simulink model "ROSCO"  (R2023a)
settings: Solver=ode4  StartTime=0.0  StopTime=TMax  FixedStep=simu.dt  RelTol=1e-3  EnableMultiTasking=on
undefined symbols (not defined in the file): A_total, Azimuth_list, B_total, Bd_total, C_total, D_total, Dd_total, DiscIntNeverNeededParam, F, n_FixFrameInputs, n_FixFrameOutputs, n_FixFrameStates2, n_RotTripletInputs, n_RotTripletOutputs, n_RotTripletStates2, new_seq_inp, new_seq_out, new_seq_states, OutList, Parameter, R, rpm2radps, simu, strmatch, uop_total, windspeed_list, wop_total, xop_total, yop_List_total
libraries: simulink x10
(part 4 of 5)

== matlab function ROSCO/LinearModel_Simulink/Switch op under Azimuth/Switch op under Azimuth ==
  data: Azimuth input; Azimuth_list input; yop_36 input; yop output
function yop  = fcn(Azimuth, Azimuth_list, yop_36)

left = 1;
right = length(Azimuth_list);

while(left<right)
    mid = floor((left + right) / 2);
    if Azimuth_list(mid) == Azimuth
        index = mid;
        break
    elseif Azimuth_list(mid) < Azimuth
        left = mid + 1;
    else
        right = mid - 1;
    end
end
% If target is not found, return the index of the interval in which it falls
if Azimuth < Azimuth_list(1)
    index = 1;
elseif Azimuth > Azimuth_list(end)
    index = length(Azimuth_list);
else
    index = left;
end

yop = yop_36(:, index);
% yop = 1/36 * yop_36(:, 1);
% for i = 2:36
%     yop = yop + 1/36 * yop_36(:, i);
% end

end

== matlab function ROSCO/Monitor2/Cyclic Pitch controller/1P Cyclic Pitch Controller1/Lead Correction ==
  data: bdq input; b_cos output size=1; psi_o input; b_sin output size=1
function [b_cos,b_sin] = fcn(bdq, psi_o)
% This block supports the Embedded MATLAB subset.
% See the help menu for details. 

b_cos=[cosd(psi_o) sind(psi_o)]*bdq;
b_sin=[-sind(psi_o) cosd(psi_o)]*bdq;

== matlab function ROSCO/LinearModel_Simulink/Transverseu/MATLAB Function ==
  data: Azimuth input; n_FixFrameInputs input; n_RotTripletInputs input; delta_u input; new_seq_inp input; delat_u_dq output
function delat_u_dq  = Transverse(Azimuth, n_FixFrameInputs, n_RotTripletInputs, delta_u, new_seq_inp)

% compute azimuth positions of blades:
az = Azimuth*pi/180.0 + 2*pi/3* (0:(3-1)) ; % Eq. 1, azimuth in radians   3个叶片的方位角（弧度），叶片1的方位角为初始方位角

% compute transformation matrices
cos_col = cos(az(:));  % 列向量
sin_col = sin(az(:));

ttv = get_tt_inverse(sin_col, cos_col);     % inverse of tt (computed analytically in function below) 逆矩阵

T1cv = zeros(n_FixFrameInputs+3*n_RotTripletInputs, n_FixFrameInputs+3*n_RotTripletInputs);

T1cv(1:n_FixFrameInputs, 1:n_FixFrameInputs) = eye(n_FixFrameInputs);                % Eq. 21  T1c的逆矩阵

for ii = 1:n_RotTripletInputs
    T1cv(n_FixFrameInputs+1+(ii-1)*3 : n_FixFrameInputs+ii*3, n_FixFrameInputs+1+(ii-1)*3 : n_FixFrameInputs+ii*3) = ttv;
end


% T1o = zeros(n_FixFrameOutputs+3*n_RotTripletOutputs, n_FixFrameOutputs+3*n_RotTripletOutputs);
% 
% T1o(1:n_FixFrameOutputs, 1:n_FixFrameOutputs) = eye(n_FixFrameOutputs);              % Tlo (Eq. 23)  输出相关
% 
% for ii = 1:n_RotTripletOutputs
%     T1o(n_FixFrameOutputs+1+(ii-1)*3 : n_FixFrameOutputs+ii*3, n_FixFrameOutputs+1+(ii-1)*3 : n_FixFrameOutputs+ii*3) = tt;
% end


%% 对u进行转换

delat_u_dq = delta_u .* 0;
delat_u_dq(new_seq_inp, :) = T1cv * delta_u(new_seq_inp);

end



function [ttv] = get_tt_inverse(sin_col, cos_col)

    c1 = cos_col(1);
    c2 = cos_col(2);
    c3 = cos_col(3);
    
    s1 = sin_col(1);
    s2 = sin_col(2);
    s3 = sin_col(3);

    
    ttv = [ c2*s3 - s2*c3,  c3*s1 - s3*c1, c1*s2 - s1*c2
               s2 - s3 ,       s3 - s1,       s1 - s2
               c3 - c2 ,       c1 - c3,       c2 - c1 ] / (1.5*sqrt(3));

    return
end

== matlab function ROSCO/LinearModel_Simulink/Diff of OP ==
  data: Avg_u input; Avg_w input; delta_u output; WindSpeed input; BldPitch input; delta_w output
function [delta_u, delta_w] = fcn(Avg_u, Avg_w, WindSpeed, BldPitch)
    % 相对于工作点的偏差
    delta_u = Avg_u;
    delta_u(1) = BldPitch(1) - Avg_u(1);
    delta_u(2) = BldPitch(2) - Avg_u(2);
    delta_u(3) = BldPitch(3) - Avg_u(3);

    delta_w = Avg_w;
    delta_w(1) = WindSpeed - Avg_w(1);
    % u(9) = BldPitch(1);  
end

== matlab function ROSCO/LinearModel_Simulink/KalmanStateObserver/iMBC ==
  data: Azimuth input; x output; xdq input
function x  = iMBC(Azimuth, xdq)

% compute azimuth positions of blades:
az = Azimuth*pi/180.0 + 2*pi/3* (0:(3-1)) ; % Eq. 1, azimuth in radians   3个叶片的方位角（弧度），叶片1的方位角为初始方位角

% compute transformation matrices
cos_col = cos(az(:));  % 列向量
sin_col = sin(az(:));

tt  = [ones(3,1), cos_col, sin_col];        % Eq. 9, t_tilde

x = xdq .* 0;
x = tt * xdq;

end

== matlab function ROSCO/LinearModel_Simulink/KalmanStateObserver/MBC1 ==
  data: Azimuth input; xdq output; x1 input; x2 input; x3 input
function xdq  = MBC(Azimuth, x1, x2, x3)
x = [x1; x2; x3];
% compute azimuth positions of blades:
az = Azimuth*pi/180.0 + 2*pi/3* (0:(3-1)) ; % Eq. 1, azimuth in radians   3个叶片的方位角（弧度），叶片1的方位角为初始方位角

% compute transformation matrices
cos_col = cos(az(:));  % 列向量
sin_col = sin(az(:));

ttv = get_tt_inverse(sin_col, cos_col);     % inverse of tt (computed analytically in function below) 逆矩阵

xdq = x .* 0;
xdq = ttv * x;

end





function [ttv] = get_tt_inverse(sin_col, cos_col)

    c1 = cos_col(1);
    c2 = cos_col(2);
    c3 = cos_col(3);
    
    s1 = sin_col(1);
    s2 = sin_col(2);
    s3 = sin_col(3);

    
    ttv = [ c2*s3 - s2*c3,  c3*s1 - s3*c1, c1*s2 - s1*c2
               s2 - s3 ,       s3 - s1,       s1 - s2
               c3 - c2 ,       c1 - c3,       c2 - c1 ] / (1.5*sqrt(3));

    return
end

== matlab function ROSCO/LinearModel_Simulink/KalmanStateObserver/MBC2 ==
  data: Azimuth input; xdq output; x1 input; x2 input; x3 input
function xdq  = MBC(Azimuth, x1, x2, x3)
x = [x1; x2; x3];
% compute azimuth positions of blades:
az = Azimuth*pi/180.0 + 2*pi/3* (0:(3-1)) ; % Eq. 1, azimuth in radians   3个叶片的方位角（弧度），叶片1的方位角为初始方位角

% compute transformation matrices
cos_col = cos(az(:));  % 列向量
sin_col = sin(az(:));

ttv = get_tt_inverse(sin_col, cos_col);     % inverse of tt (computed analytically in function below) 逆矩阵

xdq = x .* 0;
xdq = ttv * x;

end





function [ttv] = get_tt_inverse(sin_col, cos_col)

    c1 = cos_col(1);
    c2 = cos_col(2);
    c3 = cos_col(3);
    
    s1 = sin_col(1);
    s2 = sin_col(2);
    s3 = sin_col(3);

    
    ttv = [ c2*s3 - s2*c3,  c3*s1 - s3*c1, c1*s2 - s1*c2
               s2 - s3 ,       s3 - s1,       s1 - s2
               c3 - c2 ,       c1 - c3,       c2 - c1 ] / (1.5*sqrt(3));

    return
end

== matlab function ROSCO/LinearModel_Simulink/KalmanStateObserver/MBC3 ==
  data: Azimuth input; xdq output; x1 input; x2 input; x3 input
function xdq  = MBC(Azimuth, x1, x2, x3)
x = [x1; x2; x3];
% compute azimuth positions of blades:
az = Azimuth*pi/180.0 + 2*pi/3* (0:(3-1)) ; % Eq. 1, azimuth in radians   3个叶片的方位角（弧度），叶片1的方位角为初始方位角

% compute transformation matrices
cos_col = cos(az(:));  % 列向量
sin_col = sin(az(:));

ttv = get_tt_inverse(sin_col, cos_col);     % inverse of tt (computed analytically in function below) 逆矩阵

xdq = x .* 0;
xdq = ttv * x;

end





function [ttv] = get_tt_inverse(sin_col, cos_col)

    c1 = cos_col(1);
    c2 = cos_col(2);
    c3 = cos_col(3);
    
    s1 = sin_col(1);
    s2 = sin_col(2);
    s3 = sin_col(3);

    
    ttv = [ c2*s3 - s2*c3,  c3*s1 - s3*c1, c1*s2 - s1*c2
               s2 - s3 ,       s3 - s1,       s1 - s2
               c3 - c2 ,       c1 - c3,       c2 - c1 ] / (1.5*sqrt(3));

    return
end

== matlab function ROSCO/LinearModel_Simulink/PredictFcn ==
  settings: updateMethod=DISCRETE
  data: x_obs input; ydq output; DT input; A input; B input; Bd input; C input; D input; Dd input; time input; Azimuth input
function ydq = PredictFcn(x_obs, DT, A, B, Bd, C, D, Dd, time, Azimuth)
    persistent Y
    persistent times
    if isempty(times)
        times = 1;
    end
    
    dt = 0.001;  % 用于Am和Bm中的原始迭代步长，需要足够小
    dt_gap = 200;  % 实际迭代步长为dt * dt_gap,即0.2s
    
    Np = 20;  % Np*dt*dt_gap的预测区间, 4s
    Nc = 5;  % Nc*dt*dt_gap的控制区间, 1s
    gaptimes = DT/(dt*dt_gap); 
    
    
    if time>=30 && isempty(Y)
        x_obs(1:17, 1) = x_obs(1:17, 1) * (dt/DT);  % 近似转化为同步长下的初始状态
        
        delta_u = zeros(3*Nc, 1);  % 旋转坐标系
        delta_u = delta_u; % 控制区间的控制量不变，控制步长为dt*dt_gap

        Tmbc  = mbc(Azimuth);

        delta_wdq = zeros(1*Np, 1);  
        delta_wdq(1, 1) = 0; % 控制区间的后续风速不变，控制步长为dt*dt_gap
    
        Am = [dt*A+eye(size(A, 1)), zeros(size(A, 1), size(C, 1));
              C, eye(size(C, 1))];
        Bm = [dt*B*Tmbc; D*Tmbc];
        Bmd = [dt*Bd; Dd];
        Cm = [zeros(size(C, 1), size(A, 1)), eye(size(C, 1))];
        
        % --------------------------计算P矩阵-----------------------------------
        P = Cm*(Am^1);
        for i = 2:Np
                P = [P; Cm*(Am^(1+dt_gap*(i-1)))];
        end
        
        % --------------------------计算H矩阵-----------------------------------
        H_c = [];
        i = 1;
        for j = 1:Nc
            if j==1
                H_c = Cm * Am^(dt_gap*(i-1)) * Bm;
            else
                if j > i
                    H_c = [H_c, zeros(size(Cm, 1), size(Bm, 2))];
                else
                    H_c = [H_c, Cm * Am^(dt_gap*(i-j)) * Bm];
                end
            end
        end
        H = H_c;
        for i = 2:Np
            H_c = [];
            for j = 1:Nc
                if j==1
                    H_c = Cm * Am^(dt_gap*(i-1)) * Bm;
                else
                    if j > i
                        H_c = [H_c, zeros(size(Cm, 1), size(Bm, 2))];
                    else
                        H_c = [H_c, Cm * Am^(dt_gap*(i-j)) * Bm];
                    end
                end
            end
            H = [H; H_c];
        end
    
        % --------------------------计算Hd矩阵-----------------------------------
        H_c = [];
        i = 1;
        for j = 1:Np
            if j==1
                H_c = Cm * Am^(dt_gap*(i-1)) * Bmd;
            else
                if j > i
                    H_c = [H_c, zeros(size(Cm, 1), size(Bmd, 2))];
                else
                    H_c = [H_c, Cm * Am^(dt_gap*(i-j)) * Bmd];
                end
            end
        end
        Hd = H_c;
        for i = 2:Np
            H_c = [];
            for j = 1:Np
                if j==1
                    H_c = Cm * Am^(dt_gap*(i-1)) * Bmd;
                else
                    if j > i
                        H_c = [H_c, zeros(size(Cm, 1), size(Bmd, 2))];
                    else
                        H_c = [H_c, Cm * Am^(dt_gap*(i-j)) * Bmd];
                    end
                end
            end
            Hd = [Hd; H_c];
        end
    
        % ----------------------------- 预测 --------------------------------
        Y_dq = P * x_obs + H * delta_u + Hd * delta_wdq;
    
        Y_dq = reshape(Y_dq, [size(C, 1), size(Y_dq, 1)/size(C, 1)]);
        % time_list = dt*(1:size(Y_dq, 2));
        
        Y = Y_dq;
        ydq = Y(:, floor(times));
        times = times + gaptimes;
    elseif ~isempty(Y) && times<Np-gaptimes
        ydq = Y(:, floor(times));
        times = times + gaptimes;
    else
        ydq = zeros(5, 1);
    end

end

function Tmbc  = mbc(Azimuth)
    % compute azimuth positions of blades:
    az = Azimuth*pi/180.0 + 2*pi/3* (0:(3-1)) ; % Eq. 1, azimuth in radians   3个叶片的方位角（弧度），叶片1的方位角为初始方位角
    
    % compute transformation matrices
    cos_col = cos(az(:));  % 列向量
    sin_col = sin(az(:));
    
    Tmbc = get_tt_inverse(sin_col, cos_col);     % inverse of tt (computed analytically in function below) 逆矩阵
end

function [ttv] = get_tt_inverse(sin_col, cos_col)
    c1 = cos_col(1);
    c2 = cos_col(2);
    c3 = cos_col(3);
    
    s1 = sin_col(1);
    s2 = sin_col(2);
    s3 = sin_col(3);

    
    ttv = [ c2*s3 - s2*c3,  c3*s1 - s3*c1, c1*s2 - s1*c2
               s2 - s3 ,       s3 - s1,       s1 - s2
               c3 - c2 ,       c1 - c3,       c2 - c1 ] / (1.5*sqrt(3));

    return
end

== matlab function ROSCO/Monitor2/Cyclic Pitch controller/1P Cyclic Pitch Controller1/d-q transformation ==
  data: RootMyb input; M_tilt output; Az input; M_yaw output; NumBl input
function [M_tilt,M_yaw] = fwdMBC2(RootMyb, Az, NumBl)
% This block supports the Embedded MATLAB subset.
% See the help menu for details.

if NumBl == 2
    
    My=RootMyb-mean(RootMyb(1:2)); %remove mean
    
    M_tilt = [cosd(Az) cosd(Az+180) 0]*My;
    M_yaw =  [sind(Az) sind(Az+180) 0]*My;
else
    My=RootMyb-mean(RootMyb); %remove mean
    
    M_tilt = [cosd(Az) cosd(Az+120) cosd(Az+240)]*My;
    M_yaw =  [sind(Az) sind(Az+120) sind(Az+240)]*My;
end

== matlab function ROSCO/Monitor2/Cyclic Pitch controller/1P Cyclic Pitch Controller1/inverse d-q transformation ==
  data: bdq input; b1 output size=1; Az input; b2 output size=1; NumBl input; b3 output size=1
function [b1,b2,b3] = bckMBC2(bdq, Az, NumBl)
% This block supports the Embedded MATLAB subset.
% See the help menu for details.


if NumBl == 2
    
    b1=[cosd(Az) sind(Az)]*bdq;
    b2=[cosd(Az - 180) sind(Az - 180)]*bdq;
    b3=0;
    
else
    b1=[cosd(Az) sind(Az)]*bdq;
    b2=[cosd(Az + 120) sind(Az + 120)]*bdq;
    b3=[cosd(Az + 240) sind(Az + 240)]*bdq;
    
end

== matlab function ROSCO/Monitor2/Cyclic Pitch controller/1P Cyclic Pitch Controller1/saturation (limit schedule)1 ==
  data: bdq_unsat input size=[2 1]; bdq output; b_avg input; M0 input; minPitch input; k output; Params input
%limit b_d and b_q so b_1,2,or3 does not get bigger than b_avg (the sinusoids don't get cut off at zero)
%unless b_avg is <0, then limit to 0
%at_limit is 1 if limited, 0 otherwise

function [bdq,k]  = fcn(bdq_unsat, b_avg, M0,minPitch,Params)

MODE    = Params(1);  % 1 no IPC below rated (no power loss), 2 IPC always on, 3 depends on mean load
M0_set  = Params(2);
k_sat   = Params(3);

if MODE == 1
    
    if (b_avg <= minPitch)
        bdq=[0;0];
        k = 0;
    else
        if (norm(bdq_unsat,2) <= b_avg - minPitch)
            bdq = bdq_unsat;
            k = 1;
        else
            bdq=bdq_unsat*((b_avg-minPitch)/norm(bdq_unsat,2));
            k = (b_avg/norm(bdq_unsat,2));
        end
    end
elseif MODE == 2
    if (norm(bdq_unsat,2) > deg2rad(15))
        bdq = bdq_unsat*(deg2rad(15)/norm(bdq_unsat,2));
        k = (deg2rad(15)/norm(bdq_unsat,2));
    else
        bdq = bdq_unsat;
        k = 1;
    end
else  % MODE 3
    if (M0 > M0_set - 1/(2*k_sat))
        if (M0 > M0_set + 1/(2*k_sat))
            bdq = bdq_unsat;
            k = 1;
        else
            k = k_sat*(M0-M0_set)+1/2;
            bdq = k*bdq_unsat;
        end
    else
        bdq = [0;0];
        k = 0;
    end
end
%
% if (b_avg <=0)
%         bdq = bdq_unsat;
% else
%     if (norm(bdq_unsat,2) <= b_avg)
%         bdq = bdq_unsat;
%     else
%         bdq = bdq_unsat;
%     end
% end

== matlab function ROSCO/Wind Speed Estimator/NaN break ==
  data: u input; y output
function y = fcn(u)

if isnan(u)
    a = 1;
end

y = u;

== matlab function ROSCO/LinearModel_Simulink/Subsystem/MATLAB Function1 ==
  data: Azimuth input; n_FixFrameInputs input; n_RotTripletInputs input; xop input; new_seq_inp input; xop_dq output
function xop_dq  = MBC_x(Azimuth, n_FixFrameInputs, n_RotTripletInputs, xop, new_seq_inp)

% compute azimuth positions of blades:
az = Azimuth*pi/180.0 + 2*pi/3* (0:(3-1)) ; % Eq. 1, azimuth in radians   3个叶片的方位角（弧度），叶片1的方位角为初始方位角

% compute transformation matrices
cos_col = cos(az(:));  % 列向量
sin_col = sin(az(:));

ttv = get_tt_inverse(sin_col, cos_col);     % inverse of tt (computed analytically in function below) 逆矩阵

T1v = zeros(2*(n_FixFrameInputs+3*n_RotTripletInputs)-1, 2*(n_FixFrameInputs+3*n_RotTripletInputs)-1);

T1v(1:n_FixFrameInputs-1, 1:n_FixFrameInputs-1) = eye(n_FixFrameInputs-1);                % Eq. 21  T1c的逆矩阵

for ii = 1:n_RotTripletInputs
    T1v(n_FixFrameInputs+(ii-1)*3 : n_FixFrameInputs-1+ii*3, n_FixFrameInputs+(ii-1)*3 : n_FixFrameInputs-1+ii*3) = ttv;
end

start = n_FixFrameInputs+3*n_RotTripletInputs;
T1v(start:start+n_FixFrameInputs-1, start:start+n_FixFrameInputs-1) = eye(n_FixFrameInputs); 
for ii = 1:n_RotTripletInputs
    T1v(start+n_FixFrameInputs+(ii-1)*3 : start+n_FixFrameInputs-1+ii*3, start+n_FixFrameInputs+(ii-1)*3 : start+n_FixFrameInputs-1+ii*3) = ttv;
end

%% 对x进行转换
xop_dq = xop .* 0;
xop_dq(new_seq_inp, :) = T1v * xop(new_seq_inp, :);

end



function [ttv] = get_tt_inverse(sin_col, cos_col)

    c1 = cos_col(1);
    c2 = cos_col(2);
    c3 = cos_col(3);
    
    s1 = sin_col(1);
    s2 = sin_col(2);
    s3 = sin_col(3);

    
    ttv = [ c2*s3 - s2*c3,  c3*s1 - s3*c1, c1*s2 - s1*c2
               s2 - s3 ,       s3 - s1,       s1 - s2
               c3 - c2 ,       c1 - c3,       c2 - c1 ] / (1.5*sqrt(3));

    return
end

== matlab function ROSCO/LinearModel_Simulink/KalmanStateObserver/Extend X_obs_Fcn2 ==
  data: QD_TFA1 input; x_k output; Q_TFA1 input; QD_TSS1 input; Q_TSS1 input; RotSpeed input; Q_BNF1 input; Q_BNE1 input; QD_BNF1 input; QD_BNE1 input
function x_k = X_obs_Fcn1(QD_TFA1, Q_TFA1, QD_TSS1, Q_TSS1, RotSpeed, Q_BNF1, Q_BNE1, QD_BNF1, QD_BNE1)
    x_k = zeros(17, 1);
    x_k(9, 1) = QD_TFA1;
    x_k(1, 1) = Q_TFA1;
    x_k(10, 1) = QD_TSS1;
    x_k(2, 1) = Q_TSS1;
    x_k(11, 1) = RotSpeed;
    x_k(3:5, 1) = Q_BNF1;
    x_k(6:8, 1) = Q_BNE1;
    x_k(12:14, 1) = QD_BNF1;
    x_k(15:17, 1) = QD_BNE1;    
end

== matlab function ROSCO/LinearModel_Simulink/LinearWT_Fcn ==
  settings: updateMethod=DISCRETE
  data: time input; delta_ydq output; delta_xop_dq input; uop_dq input; A input; B input; C input; D input; DT input
function delta_ydq = LWT_Fcn(time, delta_xop_dq, uop_dq, A, B, C, D, DT)
    persistent delta_y_dq
    persistent times
    if isempty(times)
        times = 1;
    end
    dt = 0.001;
    Np = 10000;  % 预测时域 Np*dt
    Nc = 8000;  % 控制时域 Nc*dt

    if time>30 && isempty(delta_y_dq)
        delta_u_dq = zeros(4, Np);
        for i = 1:Np
            if i<=Nc
                delta_u_dq(:, i) = uop_dq - uop_dq;
                delta_u_dq(1, i) = 15 - 14;
            else
                delta_u_dq(:, i) = uop_dq - uop_dq;
                delta_u_dq(1, i) = 15 - 14;
                w = 0; 
            end
        end
        % 控制动作集合
        delta_y_dq = zeros(size(D, 1), Np);
        % 预测
        for i = 1:Np
            delta_xdq = delta_xop_dq;  % 初始值
            delta_xdq_dot = A * delta_xdq + B * delta_u_dq(:, i);
            delta_y_dq(:, i) = C * delta_xdq + D * delta_u_dq(:, i);
            delta_xdq = delta_xdq + dt * delta_xdq_dot;
        end

        delta_ydq = delta_y_dq(:, times);
        times = times + DT/dt;
    elseif ~isempty(delta_y_dq) && times<Np-10
        delta_ydq = delta_y_dq(:, times);
        times = times + DT/dt;  
    else
        delta_ydq = zeros(size(C, 1), 1);
    end
end

== matlab function ROSCO/LinearModel_Simulink/uop2uop_dq/MATLAB Function1 ==
  data: Azimuth input; n_FixFrameInputs input; n_RotTripletInputs input; u input; new_seq_inp input; u_dq output
function u_dq  = Transverse(Azimuth, n_FixFrameInputs, n_RotTripletInputs, u, new_seq_inp)

% compute azimuth positions of blades:
az = Azimuth*pi/180.0 + 2*pi/3* (0:(3-1)) ; % Eq. 1, azimuth in radians   3个叶片的方位角（弧度），叶片1的方位角为初始方位角

% compute transformation matrices
cos_col = cos(az(:));  % 列向量
sin_col = sin(az(:));

ttv = get_tt_inverse(sin_col, cos_col);     % inverse of tt (computed analytically in function below) 逆矩阵

T1cv = zeros(n_FixFrameInputs+3*n_RotTripletInputs, n_FixFrameInputs+3*n_RotTripletInputs);

T1cv(1:n_FixFrameInputs, 1:n_FixFrameInputs) = eye(n_FixFrameInputs);                % Eq. 21  T1c的逆矩阵

for ii = 1:n_RotTripletInputs
    T1cv(n_FixFrameInputs+1+(ii-1)*3 : n_FixFrameInputs+ii*3, n_FixFrameInputs+1+(ii-1)*3 : n_FixFrameInputs+ii*3) = ttv;
end


% T1o = zeros(n_FixFrameOutputs+3*n_RotTripletOutputs, n_FixFrameOutputs+3*n_RotTripletOutputs);
% 
% T1o(1:n_FixFrameOutputs, 1:n_FixFrameOutputs) = eye(n_FixFrameOutputs);              % Tlo (Eq. 23)  输出相关
% 
% for ii = 1:n_RotTripletOutputs
%     T1o(n_FixFrameOutputs+1+(ii-1)*3 : n_FixFrameOutputs+ii*3, n_FixFrameOutputs+1+(ii-1)*3 : n_FixFrameOutputs+ii*3) = tt;
% end


%% 对u进行转换

u_dq = u .* 0;
u_dq(new_seq_inp, :) = T1cv * u(new_seq_inp);

end



function [ttv] = get_tt_inverse(sin_col, cos_col)

    c1 = cos_col(1);
    c2 = cos_col(2);
    c3 = cos_col(3);
    
    s1 = sin_col(1);
    s2 = sin_col(2);
    s3 = sin_col(3);

    
    ttv = [ c2*s3 - s2*c3,  c3*s1 - s3*c1, c1*s2 - s1*c2
               s2 - s3 ,       s3 - s1,       s1 - s2
               c3 - c2 ,       c1 - c3,       c2 - c1 ] / (1.5*sqrt(3));

    return
end

== matlab function ROSCO/LinearModel_Simulink/Subsystem1/MATLAB Function1 ==
  data: Azimuth input; y output; n_FixFrameOutputs input; n_RotTripletOutputs input; new_seq_out input; y_dq input
function y  = iTransverse_y(Azimuth, n_FixFrameOutputs, n_RotTripletOutputs, new_seq_out, y_dq)

% compute azimuth positions of blades:
az = Azimuth*pi/180.0 + 2*pi/3* (0:(3-1)) ; % Eq. 1, azimuth in radians   3个叶片的方位角（弧度），叶片1的方位角为初始方位角

% compute transformation matrices
cos_col = cos(az(:));  % 列向量
sin_col = sin(az(:));

tt  = [ones(3,1), cos_col, sin_col];        % Eq. 9, t_tilde


T1o = zeros(n_FixFrameOutputs+3*n_RotTripletOutputs, n_FixFrameOutputs+3*n_RotTripletOutputs);

T1o(1:n_FixFrameOutputs, 1:n_FixFrameOutputs) = eye(n_FixFrameOutputs);              % Tlo (Eq. 23)  输出相关

for ii = 1:n_RotTripletOutputs
    T1o(n_FixFrameOutputs+1+(ii-1)*3 : n_FixFrameOutputs+ii*3, n_FixFrameOutputs+1+(ii-1)*3 : n_FixFrameOutputs+ii*3) = tt;
end

y = y_dq .* 0;
y(new_seq_out, :) = T1o * y_dq(new_seq_out);

end

== matlab function ROSCO/Monitor2/Cyclic Pitch controller/2P Cyclic Pitch Controller2/Lead Correction ==
  data: bdq input; b_cos output size=1; psi_o input; b_sin output size=1
function [b_cos,b_sin] = fcn(bdq, psi_o)
% This block supports the Embedded MATLAB subset.
% See the help menu for details. 

b_cos=[cosd(psi_o) sind(psi_o)]*bdq;
b_sin=[-sind(psi_o) cosd(psi_o)]*bdq;

== matlab function ROSCO/Wind Speed Estimator/MATLAB Function ==
  settings: updateMethod=DISCRETE  sampleTime=simu.dt
  data: omega_r input; tau_g input; beta input; WE_params input; A_op input; vh output; xh input; P input; K input; xh output; P output; K output; dt input; t input; HorWind input; Cx parameter; Debug output
function [vh,xh,P,K,Debug] = WSE_EKF(omega_r, tau_g, beta, WE_params, A_op, xh,P,K,dt,t,HorWind, Cx)
% This function defines a WSE based off of an Extended Kalman Filter
% Inputs:
% Outputs:
% Nikhar Abbas

% Load R variables
J       = WE_params(1);                    % Rotor Inertia
rho     = WE_params(2);                % Air density
Rr      = WE_params(3);             % Rotor Radius, R
Ng      = WE_params(4);             % Gearbox Ratio

% Simulink Offset, between mean wind speeds due to poor startup transients
sOff    = 0.8;

% Constants
H       = [1 0 0];
R       = 0.02;
L       = 6 * Rr;
Ti      = 0.2;
A       = pi*Rr^2;                         % Rotor Swept Area, m^2


% organize Inputs
if t < dt
    om_r    = omega_r;
    v_t     = 0;
    v_m     = HorWind + sOff;
else
    om_r    = xh(1);
    v_t     = xh(2);
    v_m     = xh(3) + sOff;
end

om_m    = omega_r;

% Debug Outs
Debug   = zeros(2,1);

% Find current estimated operating conditions, and saturate
v_r     = v_t + v_m;
lambda  = om_m * Rr / v_r;
lambda  = max( min(lambda, Cx.TSR(end)), Cx.TSR(1));


% A_op (system pole) interpolation
% A_op    = interp1(R.WE_FOPoles_v,R.WE_FOPoles,xh(1) + xh(2));


% Cp interpolation
Cp      = interp2(Cx.BlPitch,Cx.TSR,Cx.Cpmat,beta * rad2deg(1),lambda);
Cp      = max(0,Cp);


% Calculate Jacobians
F       = zeros(3,3);

F(1,1)      = A_op;
F(1,2)      = 1/(2*J)*rho*A*Cp*3*(v_m+v_t)^2*1/om_r;
F(1,3)      = 1/(2*J)*rho*A*Cp*3*(v_m+v_t)^2*1/om_r;

F(2,2)      = pi * v_m / (2*L);
F(2,3)      = pi * v_t / (2*L);  % this was 0


% Calculate Covariance
Q           = zeros(3,3);
Q(1,1)      = 1e-5;                     %in DZ WSE, 1e-6
Q(2,2)      = pi * v_m^3 * Ti^2 / L;
Q(3,3)      = 2^2/600;


%% Prediction Update

% states
tau_r       = 1/2 * rho * A * Cp * v_r^3 / om_m;       % Torque calculation
tau_r       = max(tau_r,0);
a           = pi * v_m / (2 * L);                           % Wind variance
dom_r       = 1/J * (tau_r - Ng * tau_g);
dv_t        = -a*v_t;
dv_m        = 0;
dxh         = [dom_r; dv_t; dv_m];

% forward euler
xh          = xh + dt*dxh;

% covariance
dP          = F*P + P*F' + Q - K*R*K';
P           = P + dt*dP;

% kalman gain
S           = H*P*H' + R;
K           = P * H' / S(1,1);   %DZ: this is odd, keep an eye on
% K           = P * H' * inv(S);   %DZ: this is odd, keep an eye on...was probably giving NJA stability issues

% output residual & update
y_til       = om_m - om_r;
xh          = xh + K*y_til;
P           = (eye(3) - K * H) * P;         % DZ: this is also different, but I think I've seen this form before


% Output Wind Speed Estimate
vh = v_m + v_t;

% Set Debug Outputs
Debug(1) = Cp;
Debug(2) = v_m;
end

== matlab function ROSCO/Monitor2/Cyclic Pitch controller/2P Cyclic Pitch Controller2/d-q transformation ==
  data: RootMyb input; M_tilt output; Az input; M_yaw output; NumBl input
function [M_tilt,M_yaw] = fwdMBC2(RootMyb, Az, NumBl)
% This block supports the Embedded MATLAB subset.
% See the help menu for details.

if NumBl == 2
    
    My=RootMyb-mean(RootMyb(1:2)); %remove mean
    
    M_tilt = [cosd(2*Az) cosd(2*(Az+180)) 0]*My;
    M_yaw =  [sind(2*Az) sind(2*(Az+180)) 0]*My;
else
    My=RootMyb-mean(RootMyb); %remove mean
    
    M_tilt = [cosd(2*Az) cosd(2*(Az+120)) cosd(2*(Az+240))]*My;
    M_yaw =  [sind(2*Az) sind(2*(Az+120)) sind(2*(Az+240))]*My;
end

== matlab function ROSCO/Monitor2/Cyclic Pitch controller/2P Cyclic Pitch Controller2/inverse d-q transformation ==
  data: bdq input; b1 output size=1; Az input; b2 output size=1; NumBl input; b3 output size=1
function [b1,b2,b3] = bckMBC2(bdq, Az, NumBl)
% This block supports the Embedded MATLAB subset.
% See the help menu for details.


if NumBl == 2
    
    b1=[cosd(2*Az) sind(2*Az)]*bdq;
    b2=[cosd(2*(Az - 180)) sind(2*(Az - 180))]*bdq;
    b3=0;
    
else
    b1=[cosd(2*Az) sind(2*Az)]*bdq;
    b2=[cosd(2*(Az + 120)) sind(2*(Az + 120))]*bdq;
    b3=[cosd(2*(Az + 240)) sind(2*(Az + 240))]*bdq;
    
end

== matlab function ROSCO/Monitor2/Cyclic Pitch controller/2P Cyclic Pitch Controller2/saturation (limit schedule)1 ==
  data: bdq_unsat input size=[2 1]; bdq output; b_avg input; M0 input; minPitch input; k output; Params input
%limit b_d and b_q so b_1,2,or3 does not get bigger than b_avg (the sinusoids don't get cut off at zero)
%unless b_avg is <0, then limit to 0
%at_limit is 1 if limited, 0 otherwise

function [bdq,k]  = fcn(bdq_unsat, b_avg, M0,minPitch,Params)

MODE    = Params(1);  % 1 no IPC below rated (no power loss), 2 IPC always on, 3
M0_set  = Params(2);
k_sat   = Params(3);

if MODE == 1
    
    if (b_avg <= minPitch)
        bdq=[0;0];
        k = 0;
    else
        if (norm(bdq_unsat,2) <= b_avg - minPitch)
            bdq = bdq_unsat;
            k = 1;
        else
            bdq=bdq_unsat*((b_avg-minPitch)/norm(bdq_unsat,2));
            k = (b_avg/norm(bdq_unsat,2));
        end
    end
elseif MODE == 2
    if (norm(bdq_unsat,2) > deg2rad(15))
        bdq = bdq_unsat*(deg2rad(15)/norm(bdq_unsat,2));
        k = (deg2rad(15)/norm(bdq_unsat,2));
    else
        bdq = bdq_unsat;
        k = 1;
    end
else  % MODE 3
    if (M0 > M0_set - 1/(2*k_sat))
        if (M0 > M0_set + 1/(2*k_sat))
            bdq = bdq_unsat;
            k = 1;
        else
            k = k_sat*(M0-M0_set)+1/2;
            bdq = k*bdq_unsat;
        end
    else
        bdq = [0;0];
        k = 0;
    end
end
%
% if (b_avg <=0)
%         bdq = bdq_unsat;
% else
%     if (norm(bdq_unsat,2) <= b_avg)
%         bdq = bdq_unsat;
%     else
%         bdq = bdq_unsat;
%     end
% end

== matlab function ROSCO/LinearModel_Simulink/Subsystem2/MATLAB Function1 ==
  data: Azimuth input; y output; n_FixFrameOutputs input; n_RotTripletOutputs input; new_seq_out input; y_dq input
function y  = iTransverse_y(Azimuth, n_FixFrameOutputs, n_RotTripletOutputs, new_seq_out, y_dq)

% compute azimuth positions of blades:
az = Azimuth*pi/180.0 + 2*pi/3* (0:(3-1)) ; % Eq. 1, azimuth in radians   3个叶片的方位角（弧度），叶片1的方位角为初始方位角

% compute transformation matrices
cos_col = cos(az(:));  % 列向量
sin_col = sin(az(:));

tt  = [ones(3,1), cos_col, sin_col];        % Eq. 9, t_tilde


T1o = zeros(n_FixFrameOutputs+3*n_RotTripletOutputs, n_FixFrameOutputs+3*n_RotTripletOutputs);

T1o(1:n_FixFrameOutputs, 1:n_FixFrameOutputs) = eye(n_FixFrameOutputs);              % Tlo (Eq. 23)  输出相关

for ii = 1:n_RotTripletOutputs
    T1o(n_FixFrameOutputs+1+(ii-1)*3 : n_FixFrameOutputs+ii*3, n_FixFrameOutputs+1+(ii-1)*3 : n_FixFrameOutputs+ii*3) = tt;
end

y = y_dq .* 0;
y(new_seq_out, :) = T1o * y_dq(new_seq_out);

end

== matlab function ROSCO/MPC/Diff of OP ==
  data: Avg_u input; Avg_w input; delta_u output; WindSpeed input; BldPitch input; delta_w output
function [delta_u, delta_w] = fcn(Avg_u, Avg_w, WindSpeed, BldPitch)
    % 相对于工作点的偏差
    delta_u = Avg_u;
    delta_u(1) = BldPitch(1) - Avg_u(1);
    delta_u(2) = BldPitch(2) - Avg_u(2);
    delta_u(3) = BldPitch(3) - Avg_u(3);

    delta_w = Avg_w;
    delta_w(1) = WindSpeed - Avg_w(1);
    % u(9) = BldPitch(1);  
end

== matlab function ROSCO/MPC/KalmanStateObserver/Extend AB ==
  settings: updateMethod=DISCRETE
  data: A input; Am output; B input; C input; D input; delta_udq_in input; Bm output; Bmd output; delta_udq output; DT input; delta_wdq_in input; Bd input; Dd input; delta_wdq output
function [Am, Bm, Bmd, delta_udq, delta_wdq] = fcn(A, B, C, D, delta_udq_in, DT, delta_wdq_in, Bd, Dd )
    persistent delta_udq_in_prior
    persistent delta_wdq_in_prior
    
    if isempty(delta_udq_in_prior)
        delta_udq_in_prior = delta_udq_in;
        delta_wdq_in_prior = delta_wdq_in;
    end
    delta_udq = delta_udq_in - delta_udq_in_prior;
    delta_wdq = delta_wdq_in - delta_wdq_in_prior;
    
    dt = 0.001;
    Am = [dt * A + eye(size(A, 1)), zeros(size(A, 1), size(C, 1));
          C, eye(size(C, 1))];
    Bm = [dt * B; D];
    Bmd = [dt * Bd; Dd];
    
    % ------------------------
    delta_udq_in_prior = delta_udq_in;
    delta_wdq_in_prior = delta_wdq_in;
end

== matlab function ROSCO/MPC/KalmanStateObserver/Extend X_obs_Fcn ==
  settings: updateMethod=DISCRETE
  data: QD_TFA1 input; X_obs output; Q_TFA1 input; QD_TSS1 input; Q_TSS1 input; RotSpeed input; ydq input
function X_obs = X_obs_Fcn(QD_TFA1, Q_TFA1, QD_TSS1, Q_TSS1, RotSpeed, ydq)
    % 需要对x进行MBC变换，但由于观测量都处于固定坐标系中，故无需进行变换
    % X为增广状态，参考文献"基于模型预测控制的大型海上风电机组降载控制"4.4.1节公式(4-28)
    persistent x_km1
    if isempty(x_km1)
        x_km1 = zeros(17, 1);
        x_km1(9, 1) = QD_TFA1;
        x_km1(1, 1) = Q_TFA1;
        x_km1(10, 1) = QD_TSS1;
        x_km1(2, 1) = Q_TSS1;
        x_km1(11, 1) = RotSpeed;
    end
    
    x_k = zeros(17, 1);
    x_k(9, 1) = QD_TFA1;
    x_k(1, 1) = Q_TFA1;
    x_k(10, 1) = QD_TSS1;
    x_k(2, 1) = Q_TSS1;
    x_k(11, 1) = RotSpeed;
    
    % 计算差分量
    delta_x_k = zeros(17, 1);
    delta_x_k(9, 1) = x_k(9, 1) - x_km1(9, 1);
    delta_x_k(1, 1) = x_k(1, 1) - x_km1(1, 1);
    delta_x_k(10, 1) = x_k(10, 1) - x_km1(10, 1);
    delta_x_k(2, 1) = x_k(2, 1) - x_km1(2, 1);
    delta_x_k(11, 1) = x_k(11, 1) - x_km1(11, 1);
    
    % 生成增广状态变量
    X_obs = zeros(17+5, 1);
    X_obs(1:17, 1) = delta_x_k;
    X_obs(18:22, 1) = ydq;

    % ----------------
    x_km1(9, 1) = x_k(9, 1);
    x_km1(1, 1) = x_k(1, 1);
    x_km1(10, 1) = x_k(10, 1);
    x_km1(2, 1) = x_k(2, 1);
    x_km1(11, 1) = x_k(11, 1);

    

end

== matlab function ROSCO/MPC/KalmanStateObserver/Extend X_obs_Fcn1 ==
  settings: updateMethod=DISCRETE
  data: QD_TFA1 input; X_obs output; Q_TFA1 input; QD_TSS1 input; Q_TSS1 input; RotSpeed input; Q_BNF1 input; Q_BNE1 input; QD_BNF1 input; QD_BNE1 input; ydq input
function X_obs = X_obs_Fcn1(QD_TFA1, Q_TFA1, QD_TSS1, Q_TSS1, RotSpeed, Q_BNF1, Q_BNE1, QD_BNF1, QD_BNE1, ydq)
    % 需要对x进行MBC变换，但由于观测量都处于固定坐标系中，故无需进行变换
    % X为增广状态，参考文献"基于模型预测控制的大型海上风电机组降载控制"4.4.1节公式(4-28)
    persistent x_km1
    if isempty(x_km1)
        x_km1 = zeros(17, 1);
        x_km1(9, 1) = QD_TFA1;
        x_km1(1, 1) = Q_TFA1;
        x_km1(10, 1) = QD_TSS1;
        x_km1(2, 1) = Q_TSS1;
        x_km1(11, 1) = RotSpeed;
        x_km1(3:5, 1) = Q_BNF1;
        x_km1(6:8, 1) = Q_BNE1;
        x_km1(12:14, 1) = QD_BNF1;
        x_km1(15:17, 1) = QD_BNE1;
    end
    
    x_k = zeros(17, 1);
    x_k(9, 1) = QD_TFA1;
    x_k(1, 1) = Q_TFA1;
    x_k(10, 1) = QD_TSS1;
    x_k(2, 1) = Q_TSS1;
    x_k(11, 1) = RotSpeed;
    x_k(3:5, 1) = Q_BNF1;
    x_k(6:8, 1) = Q_BNE1;
    x_k(12:14, 1) = QD_BNF1;
    x_k(15:17, 1) = QD_BNE1;
    
    % 计算差分量
    delta_x_k = zeros(17, 1);
    delta_x_k(9, 1) = x_k(9, 1) - x_km1(9, 1);
    delta_x_k(1, 1) = x_k(1, 1) - x_km1(1, 1);
    delta_x_k(10, 1) = x_k(10, 1) - x_km1(10, 1);
    delta_x_k(2, 1) = x_k(2, 1) - x_km1(2, 1);
    delta_x_k(11, 1) = x_k(11, 1) - x_km1(11, 1);
    delta_x_k(3:5, 1) = x_k(3:5, 1) - x_km1(3:5, 1);
    delta_x_k(6:8, 1) = x_k(6:8, 1) - x_km1(6:8, 1);
    delta_x_k(12:14, 1) = x_k(12:14, 1) - x_km1(12:14, 1);
    delta_x_k(15:17, 1) = x_k(15:17, 1) - x_km1(15:17, 1);
    
    % 生成增广状态变量
    X_obs = zeros(17+5, 1);
    X_obs(1:17, 1) = delta_x_k;
    X_obs(18:22, 1) = ydq;

    % ----------------
    x_km1(9, 1) = x_k(9, 1);
    x_km1(1, 1) = x_k(1, 1);
    x_km1(10, 1) = x_k(10, 1);
    x_km1(2, 1) = x_k(2, 1);
    x_km1(11, 1) = x_k(11, 1);
    x_km1(3:5, 1) = x_k(3:5, 1);
    x_km1(6:8, 1) = x_k(6:8, 1);
    x_km1(12:14, 1) = x_k(12:14, 1);
    x_km1(15:17, 1) = x_k(15:17, 1);
    

end

== matlab function ROSCO/MPC/KalmanStateObserver/Extend X_obs_Fcn2 ==
  data: QD_TFA1 input; x_k output; Q_TFA1 input; QD_TSS1 input; Q_TSS1 input; RotSpeed input; Q_BNF1 input; Q_BNE1 input; QD_BNF1 input; QD_BNE1 input
function x_k = X_obs_Fcn1(QD_TFA1, Q_TFA1, QD_TSS1, Q_TSS1, RotSpeed, Q_BNF1, Q_BNE1, QD_BNF1, QD_BNE1)
    x_k = zeros(17, 1);
    x_k(9, 1) = QD_TFA1;
    x_k(1, 1) = Q_TFA1;
    x_k(10, 1) = QD_TSS1;
    x_k(2, 1) = Q_TSS1;
    x_k(11, 1) = RotSpeed;
    x_k(3:5, 1) = Q_BNF1;
    x_k(6:8, 1) = Q_BNE1;
    x_k(12:14, 1) = QD_BNF1;
    x_k(15:17, 1) = QD_BNE1;    
end

== matlab function ROSCO/MPC/KalmanStateObserver/KalmanSP ==
  data: Am input; X_pred output; Bm input; Bmd input; X_obs input; delta_udq input; delta_wdq input
function X_pred = KalmanSP(Am, Bm, Bmd, X_obs, delta_udq, delta_wdq)
    persistent x_hat
    persistent P

    if isempty(x_hat)
        x_hat = zeros(22, 1);
        P = eye(22);
    end

    H = zeros(22, 22);  % 量测状态矩阵
    % 选择可量测量
    H(1, 1) = 1; 
    H(2, 2) = 1; 
    H(9, 9) = 1;
    H(10, 10) = 1;
    H(11, 11) = 1;
    H(18, 18) = 1;  % GenSpeed
    H(19, 19) = 1;  % RotSpeed


    Q = 1 * eye(22);     % 过程噪声协方差矩阵
    Q(20, 20) = 100;
    Q(21, 21) = 100;
    Q(22, 22) = 100;
    R = 1e-8 * eye(22);  % 观测噪声协方差
    
    v = sqrt(R) * ones(22, 1) * randn;
    z  = H * X_obs + v;
    
    % 时间更新（预测）
    x_hat_ = Am * x_hat + Bm * delta_udq + Bmd * delta_wdq;
    P_ = Am * P * Am' + Q;

    % 测量更新（校正）
    K = P_ * H' * (H * P_ * H' + R)^(-1);
    P = (eye(22) - K * H) * P_;

    x_hat = x_hat_ + K * (z - H * x_hat_);

    X_pred = x_hat;



end

== matlab function ROSCO/MPC/KalmanStateObserver/MATLAB Function1 ==
  data: Azimuth input; ydq output; n_FixFrameOutputs input; n_RotTripletOutputs input; new_seq_out input; y input
function ydq  = Transverse_y(Azimuth, n_FixFrameOutputs, n_RotTripletOutputs, new_seq_out, y)

% compute azimuth positions of blades:
az = Azimuth*pi/180.0 + 2*pi/3* (0:(3-1)) ; % Eq. 1, azimuth in radians   3个叶片的方位角（弧度），叶片1的方位角为初始方位角

% compute transformation matrices
cos_col = cos(az(:));  % 列向量
sin_col = sin(az(:));

ttv = get_tt_inverse(sin_col, cos_col);     % inverse of tt (computed analytically in function below) 逆矩阵

T1ov = zeros(n_FixFrameOutputs+3*n_RotTripletOutputs, n_FixFrameOutputs+3*n_RotTripletOutputs);

T1ov(1:n_FixFrameOutputs, 1:n_FixFrameOutputs) = eye(n_FixFrameOutputs);              % Tlo (Eq. 23)  输出相关

for ii = 1:n_RotTripletOutputs
    T1ov(n_FixFrameOutputs+1+(ii-1)*3 : n_FixFrameOutputs+ii*3, n_FixFrameOutputs+1+(ii-1)*3 : n_FixFrameOutputs+ii*3) = ttv;
end

ydq = y .* 0;
ydq(new_seq_out, :) = T1ov * y(new_seq_out);

end





function [ttv] = get_tt_inverse(sin_col, cos_col)

    c1 = cos_col(1);
    c2 = cos_col(2);
    c3 = cos_col(3);
    
    s1 = sin_col(1);
    s2 = sin_col(2);
    s3 = sin_col(3);

    
    ttv = [ c2*s3 - s2*c3,  c3*s1 - s3*c1, c1*s2 - s1*c2
               s2 - s3 ,       s3 - s1,       s1 - s2
               c3 - c2 ,       c1 - c3,       c2 - c1 ] / (1.5*sqrt(3));

    return
end

== matlab function ROSCO/MPC/KalmanStateObserver/MBC ==
  data: Azimuth input; xdq output; x1 input; x2 input; x3 input
function xdq  = MBC(Azimuth, x1, x2, x3)
x = [x1; x2; x3];
% compute azimuth positions of blades:
az = Azimuth*pi/180.0 + 2*pi/3* (0:(3-1)) ; % Eq. 1, azimuth in radians   3个叶片的方位角（弧度），叶片1的方位角为初始方位角

% compute transformation matrices
cos_col = cos(az(:));  % 列向量
sin_col = sin(az(:));

ttv = get_tt_inverse(sin_col, cos_col);     % inverse of tt (computed analytically in function below) 逆矩阵

xdq = x .* 0;
xdq = ttv * x;

end





function [ttv] = get_tt_inverse(sin_col, cos_col)

    c1 = cos_col(1);
    c2 = cos_col(2);
    c3 = cos_col(3);
    
    s1 = sin_col(1);
    s2 = sin_col(2);
    s3 = sin_col(3);

    
    ttv = [ c2*s3 - s2*c3,  c3*s1 - s3*c1, c1*s2 - s1*c2
               s2 - s3 ,       s3 - s1,       s1 - s2
               c3 - c2 ,       c1 - c3,       c2 - c1 ] / (1.5*sqrt(3));

    return
end

== matlab function ROSCO/MPC/KalmanStateObserver/MBC1 ==
  data: Azimuth input; xdq output; x1 input; x2 input; x3 input
function xdq  = MBC(Azimuth, x1, x2, x3)
x = [x1; x2; x3];
% compute azimuth positions of blades:
az = Azimuth*pi/180.0 + 2*pi/3* (0:(3-1)) ; % Eq. 1, azimuth in radians   3个叶片的方位角（弧度），叶片1的方位角为初始方位角

% compute transformation matrices
cos_col = cos(az(:));  % 列向量
sin_col = sin(az(:));

ttv = get_tt_inverse(sin_col, cos_col);     % inverse of tt (computed analytically in function below) 逆矩阵

xdq = x .* 0;
xdq = ttv * x;

end





function [ttv] = get_tt_inverse(sin_col, cos_col)

    c1 = cos_col(1);
    c2 = cos_col(2);
    c3 = cos_col(3);
    
    s1 = sin_col(1);
    s2 = sin_col(2);
    s3 = sin_col(3);

    
    ttv = [ c2*s3 - s2*c3,  c3*s1 - s3*c1, c1*s2 - s1*c2
               s2 - s3 ,       s3 - s1,       s1 - s2
               c3 - c2 ,       c1 - c3,       c2 - c1 ] / (1.5*sqrt(3));

    return
end

== matlab function ROSCO/MPC/KalmanStateObserver/MBC2 ==
  data: Azimuth input; xdq output; x1 input; x2 input; x3 input
function xdq  = MBC(Azimuth, x1, x2, x3)
x = [x1; x2; x3];
% compute azimuth positions of blades:
az = Azimuth*pi/180.0 + 2*pi/3* (0:(3-1)) ; % Eq. 1, azimuth in radians   3个叶片的方位角（弧度），叶片1的方位角为初始方位角

% compute transformation matrices
cos_col = cos(az(:));  % 列向量
sin_col = sin(az(:));

ttv = get_tt_inverse(sin_col, cos_col);     % inverse of tt (computed analytically in function below) 逆矩阵

xdq = x .* 0;
xdq = ttv * x;

end





function [ttv] = get_tt_inverse(sin_col, cos_col)

    c1 = cos_col(1);
    c2 = cos_col(2);
    c3 = cos_col(3);
    
    s1 = sin_col(1);
    s2 = sin_col(2);
    s3 = sin_col(3);

    
    ttv = [ c2*s3 - s2*c3,  c3*s1 - s3*c1, c1*s2 - s1*c2
               s2 - s3 ,       s3 - s1,       s1 - s2
               c3 - c2 ,       c1 - c3,       c2 - c1 ] / (1.5*sqrt(3));

    return
end

== matlab function ROSCO/MPC/KalmanStateObserver/MBC3 ==
  data: Azimuth input; xdq output; x1 input; x2 input; x3 input
function xdq  = MBC(Azimuth, x1, x2, x3)
x = [x1; x2; x3];
% compute azimuth positions of blades:
az = Azimuth*pi/180.0 + 2*pi/3* (0:(3-1)) ; % Eq. 1, azimuth in radians   3个叶片的方位角（弧度），叶片1的方位角为初始方位角

% compute transformation matrices
cos_col = cos(az(:));  % 列向量
sin_col = sin(az(:));

ttv = get_tt_inverse(sin_col, cos_col);     % inverse of tt (computed analytically in function below) 逆矩阵

xdq = x .* 0;
xdq = ttv * x;

end





function [ttv] = get_tt_inverse(sin_col, cos_col)

    c1 = cos_col(1);
    c2 = cos_col(2);
    c3 = cos_col(3);
    
    s1 = sin_col(1);
    s2 = sin_col(2);
    s3 = sin_col(3);

    
    ttv = [ c2*s3 - s2*c3,  c3*s1 - s3*c1, c1*s2 - s1*c2
               s2 - s3 ,       s3 - s1,       s1 - s2
               c3 - c2 ,       c1 - c3,       c2 - c1 ] / (1.5*sqrt(3));

    return
end

== matlab function ROSCO/MPC/KalmanStateObserver/iMBC ==
  data: Azimuth input; x output; xdq input
function x  = iMBC(Azimuth, xdq)

% compute azimuth positions of blades:
az = Azimuth*pi/180.0 + 2*pi/3* (0:(3-1)) ; % Eq. 1, azimuth in radians   3个叶片的方位角（弧度），叶片1的方位角为初始方位角

% compute transformation matrices
cos_col = cos(az(:));  % 列向量
sin_col = sin(az(:));

tt  = [ones(3,1), cos_col, sin_col];        % Eq. 9, t_tilde

x = xdq .* 0;
x = tt * xdq;

end

== matlab function ROSCO/MPC/MPC ==
  settings: updateMethod=DISCRETE
  data: simu_dt input; u_next output; delta_w_list input; Rs_1 input; xobs_dq input; u_init input; Azimuth input; RotSpeed input; A input; B input; C input; D input; Bd input; Dd input
function u_next = MPC(simu_dt, delta_w_list, Rs_1, xobs_dq, u_init, Azimuth, RotSpeed, A, B, C, D, Bd, Dd)
    persistent sn
    persistent u_hold
    persistent u_hold_pre
    if isempty(sn)
        sn = 1;
        u_hold = u_init .* 0;
        u_hold_pre = u_hold;
    end
    % 定义步长相关变量
    DT = 1e-3;  % 积分步长，一定要足够小，不然积分会发散
    DT_gap = 100; % 实际步长为DT*DT_gap
    Np = 20;
    Nc = 5;
    %% MPC生成控制量
    if rem(sn, (DT/simu_dt)*DT_gap)==1
        % --------------------------- 设置当前时刻的输入量 -----------------------
        % ------------------------------- 风速序列 -------------------------------
        %delta_w_list 
        % -------------------------- 设置参考输出序列 ----------------------------
        %Rs_1 = [1173.6; 12.1; 5700; 0; 0]; 
        Rs = zeros(5*Np, 1);  % Rs_1中第三个值需要根据工作点来选
        for ii = 1:Np
            Rs(1+5*(ii-1):5*ii, 1) = Rs_1;
        end

        % --------------------------- 设置输出权重 ------------------------------
        Q_1 = eye(5); Q = eye(5*Np);
        Q_1(1, 1) = 6*1e4; Q_1(2, 2) = 0; Q_1(3, 3) = 0; Q_1(4, 4) = 1000; Q_1(5, 5) = 1000; 
        for ii = 1:Np
            Q(1+5*(ii-1):5*ii, 1+5*(ii-1):5*ii) = Q_1;
        end
        % -------------------------- 设置输入权重 -----------------------------
        R_1 = 1e13 * eye(3); R = eye(3*Nc);
        for ii = 1:Nc
            R(1+3*(ii-1):3*ii, 1+3*(ii-1):3*ii) = R_1;
        end

        % 当前步的初始状态和控制动作
        % ------------------------------- 当前状态 ---------------------------------------
        xdq_k = xobs_dq;   % [delta_xdq_dot; y_dq]
        xdq_k(1:17, 1) = xdq_k(1:17, 1) * (DT/simu_dt);  % 近似转化为同步长下的初始状态
        % u_init % 初始控制动作(旋转坐标系)


        %% --------------------------- 求解下一步的控制量 -----------------------
        u_hold_pre = u_hold;
        u_hold = MPC_Step(A, B, C, D, Bd, Dd, xdq_k, u_init, Np, Nc, DT, DT_gap, delta_w_list, Rs, Q, R, Azimuth, RotSpeed);
        
        u_next = u_hold_pre + 1/((DT/simu_dt)*DT_gap)*(u_hold - u_hold_pre);
        % delta_u = u_next - uop; % 相比于工作点的增量
        % 理论上，要减小叶根弯矩，需要增大桨距角
    else
        if rem(sn, (DT/simu_dt)*DT_gap)==0
            u_next = u_hold;
        else
            u_next = u_hold_pre + rem(sn, (DT/simu_dt)*DT_gap)/((DT/simu_dt)*DT_gap)*(u_hold - u_hold_pre);  % 插值或对输出加一个一阶惯性环节，目的是平滑控制信号的输出
        end
    end
    sn = sn + 1;

end


function u_next = MPC_Step(A, B, C, D, Bd, Dd, xdq_init, u_init, Np, Nc, DT, DT_gap, delta_w_list, Rs, Q, R, Azimuth, RotSpeed)
    
    %% 差分方程的矩阵
    Am = [DT*A+eye(size(A, 1)), zeros(size(A, 1), size(C, 1));
          C, eye(size(C, 1))];
    Bm = [DT*B; D];
    Bmd = [DT*Bd; Dd];
    Cm = [zeros(size(C, 1), size(A, 1)), eye(size(C, 1))];
    
    %% 预测方程的矩阵
    % 计算矩阵Timbc
    % M = eye(size(D, 1));
    % M(3:5, 3:5) = imbc_in;
    % Timbc = zeros(size(D, 1)*Np, size(D, 1)*Np);
    % for i = 1:Np
    %     Timbc(1+size(D, 1)*(i-1):size(D, 1)*i, 1+size(D, 1)*(i-1):size(D, 1)*i) = M;
    % end
    % ---------------------------------- 计算矩阵P ----------------------------
    P = [];
    for i = 1:Np
        if i == 1
            P = Cm*(Am^1);
        else
            P = [P; Cm*(Am^(1+DT_gap*(i-1)))];
        end
    end
    % P = Timbc * P;
    % ---------------------------------- 计算矩阵H ----------------------------
    Azimuth_list = Azimuth * ones(1, Nc);
    for i = 2:Nc
        Azimuth_list(i) = rem(Azimuth_list(i-1) + rad2deg(RotSpeed * DT * DT_gap), 360);
    end
    

    H = [];
    for i = 1:Np
        H_c = [];
        for j = 1:Nc
            if j==1
                H_c = Cm * Am^(DT_gap*(i-1)) * Bm * mbc(Azimuth_list(j));
            else
                if j > i
                    H_c = [H_c, zeros(size(Cm, 1), size(Bm, 2))];
                else
                    H_c = [H_c, Cm * Am^(DT_gap*(i-j)) * Bm * mbc(Azimuth_list(j))];
                end
            end
        end
        if i == 1
            H = H_c;
        else
            H = [H; H_c];
        end
    end
    % H = Timbc*H;
    % ---------------------------------- 计算矩阵Hd ----------------------------
    Hd = [];
    for i = 1:Np
        H_c = [];
        for j = 1:Np
            if j==1
                H_c = Cm * Am^(DT_gap*(i-1)) * Bmd;
            else
                if j > i
                    H_c = [H_c, zeros(size(Cm, 1), size(Bmd, 2))];
                else
                    H_c = [H_c, Cm * Am^(DT_gap*(i-j)) * Bmd];
                end
            end
        end
        if i == 1
            Hd = H_c;
        else
            Hd = [Hd; H_c];
        end
    end
    % Hd = Timbc*Hd;
    %% ------------------------------- 求解最优控制序列 ---------------------------------------
    % 控制输入的约束
    delta_u_max = [2; 2; 2] * (pi / 180) * (DT * DT_gap); % 变桨速率约束的上限 rad
    delta_u_min = delta_u_max; % 变桨速率约束的下限 rad
    u_max = [90; 90; 90] * (pi / 180); % 变桨约束上限 rad
    u_min = [0; 0; 0] * (pi / 180); % 变桨约束下限 rad
    % 构造二次型的矩阵
    % E
    E = H' * Q * H + R;
    % F
    F = 2 * (P * xdq_init + Hd * delta_w_list - Rs)' * Q * H;
    % 约束相关矩阵
    b = zeros(4*Nc*3, 1);
    for i = 1:Nc
        b(1+3*(i-1):3*i, 1) = delta_u_max;
    end
    for i = 1:Nc
        b(1+3*Nc+3*(i-1):3*Nc+3*i, 1) = delta_u_min;
    end
    for i = 1:Nc
        b(1+6*Nc+3*(i-1):6*Nc+3*i, 1) = u_max-u_init;
    end
    for i = 1:Nc
        b(1+9*Nc+3*(i-1):9*Nc+3*i, 1) = u_min+u_init;
    end
    % Acons
    Acons = zeros(12*Nc, 3*Nc);
    Acons(1:3*Nc, :) = eye(3*Nc);
    Acons(1+3*Nc:6*Nc, :) = -1*eye(3*Nc);
    K = zeros(3*Nc, 3*Nc);
    for i = 1:Nc
        for j = 1:Nc
            if i>=j
                K(1+3*(i-1):3*i, 1+3*(j-1):3*j) = eye(3);
            end
        end
    end
    Acons(1+6*Nc:9*Nc, :) = K;
    Acons(1+9*Nc:12*Nc, :) = -1 * K;
    % 得到二次型优化问题
    % J = delta_u_list' * E * delta_u_list + F * delta_u_list
    % Acons * delta_u_list <= b
    options = optimoptions('quadprog','MaxIterations', 1000, 'Display','off', 'Algorithm', 'active-set');
    Aeq = [];
    beq = [];
    lb = [];
    ub = [];
    x0 = zeros(size(u_init, 1)*Nc, 1);
    [delta_u_list, ~, exitflag] = quadprog(E, F', Acons, b, Aeq,beq,lb,ub,x0,options);
    if exitflag == 1
        % 正常解
        u_next = delta_u_list(1:3, 1) + u_init;
    else
        u_next = u_init;
    end

end



function Tmbc  = mbc(Azimuth)
    % compute azimuth positions of blades:
    az = Azimuth*pi/180.0 + 2*pi/3* (0:(3-1)) ; % Eq. 1, azimuth in radians   3个叶片的方位角（弧度），叶片1的方位角为初始方位角
    
    % compute transformation matrices
    cos_col = cos(az(:));  % 列向量
    sin_col = sin(az(:));
    
    Tmbc = get_tt_inverse(sin_col, cos_col);     % inverse of tt (computed analytically in function below) 逆矩阵
end

function Timbc = imbc(Azimuth)
    az = Azimuth*pi/180.0 + 2*pi/3* (0:(3-1)) ; % Eq. 1, azimuth in radians   3个叶片的方位角（弧度），叶片1的方位角为初始方位角
    
    % compute transformation matrices
    cos_col = cos(az(:));  % 列向量
    sin_col = sin(az(:));
    
    Timbc  = [ones(3,1), cos_col, sin_col];        % Eq. 9, t_tilde
end

function [ttv] = get_tt_inverse(sin_col, cos_col)
    c1 = cos_col(1);
    c2 = cos_col(2);
    c3 = cos_col(3);
    
    s1 = sin_col(1);
    s2 = sin_col(2);
    s3 = sin_col(3);

    
    ttv = [ c2*s3 - s2*c3,  c3*s1 - s3*c1, c1*s2 - s1*c2
               s2 - s3 ,       s3 - s1,       s1 - s2
               c3 - c2 ,       c1 - c3,       c2 - c1 ] / (1.5*sqrt(3));

    return
end

== matlab function ROSCO/MPC/Reference Generate ==
  data: WindSpeed input; Rs_1 output
function Rs_1 = fcn(WindSpeed)
    Rs_1 = [1173.6; 12.1; 6300; 0; 0];   % 独立变桨需要最小化第4,5变量，即M_tilt和M_yaw
end
